simulink model "RTex"  (Simulink 10.0)
settings: Solver=ode3  StartTime=0.0  StopTime=inf  FixedStep=0.05  RelTol=1e-3  EnableMultiTasking=on
settings Model: Creator=unknown  LastModifiedBy=unknown  SimulationMode=external  ExtModeTrigMode=oneshot  ExtModeArmWhenConnect=off
settings DataIOCC: SignalLoggingSaveFormat=ModelDataLogs
settings OptimizationCC: BlockReduction=off  BooleanDataType=off  LocalBlockOutputs=off  InitFltsAndDblsToZero=on
settings DebuggingCC: SaveWithParameterizedLinksMsg=none  SignalResolutionControl=TryResolveAllWithWarning  MultiTaskDSMMsg=warning  MultiTaskCondExecSysMsg=none  FcnCallInpInsideContextMsg=warning
settings HardwareCC: TargetBitPerLong=64  TargetBitPerPointer=64  TargetBitPerSizeT=64  TargetBitPerPtrDiffT=64  TargetLongLongMode=on  TargetIntDivRoundTo=Zero  TargetEndianess=LittleEndian  TargetWordSize=64  TargetHWDeviceType=MATLAB Host  ProdEqTarget=off
settings SFSimCC: SimUseLocalCustomCode=on  CustomCodeUndefinedFunction=FilterOut
settings RTWCC: MakeCommand="make_rtw S_FUNCTIONS_LIB=\"..\\winmm.lib ..\\rt.lib\""  RetainRTWFile=on  RTWUseLocalCustomCode=on
settings GRTTargetCC: TargetFcnLib=ansi_tfl_tmw.mat  ExtMode=on

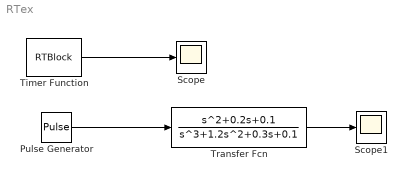
== system RTex ==
  Pulse Generator : DiscretePulseGenerator  PulseType=Time based  Period=1  PulseWidth=50
  Scope : Scope
  Scope1 : Scope
  Timer Function : S-Function  FunctionName=RTBlock  Parameters=step,priority,ThPriority  SFunctionDeploymentMode=off  EnableBusSupport=off  mask(RTBlock){step=50, priority=HIGH, ThPriority=TIME CRITICAL}
      mask prompts: step "Timestep (ms)"; ThPriority "Thread Priority"
      mask help:
      | Real Time Block: Set the characteristics of a real-time simulation. The settings of the simulation are selectable using the block panel. The parameters are:
      |
      | - Timeout: in milliseconds, defines the temporization with which Simulink requires to the Operating System the availability of resources for the execution of the simulation step. The value should be fixed equal to the simulation step of Simulink (the timestep);
      |
      | - Priority Class: defines the class of task priority required, that can be one of the following values:
      | -- IDLE PRIORITY: Low priority, typical of an idle process (priority less than normal)
      | -- NORMAL PRIORITY: Typical priority of a typical windows application;
      | -- HIGH PRIORITY: Typical priority of a relevant application, that needs more resources of a normal application;
      | -- REAL-TIME PRIORITY: Exclusive priority of a unique process that needs all the resources of the operating system.
      |
      | - Thread Priority: defines the class of task priority required, that can be one of the following values:
      | -- IDLE : The thread should run when the main process is inactive.
      | -- LOWEST : The thread runs with a minimal respect of the temporization;
      | -- NORMAL : The thread runs with the same priority of the main process;
      | -- HIGH : The thread runs with the major priority respect to the main process;
      | -- REAL-TIME : The process runs when the simulation thread is in idle state.
      mask TypeOptions priority: IDLE | NORMAL | HIGH | REAL-TIME
      mask TypeOptions ThPriority: IDLE | LOWEST | NORMAL | HIGHEST | TIME CRITICAL
  Transfer Fcn : TransferFcn  Numerator=[1 0.2 0.1]  Denominator=[1 1.2 0.3 0.1]
  wires:
  Timer Function/1 -> Scope/1
  Pulse Generator/1 -> Transfer Fcn/1
  Transfer Fcn/1 -> Scope1/1
